simulink model "simulink_Cartpend_noControl"  (R2015a)
settings: Solver=ode45  StartTime=0.0  StopTime=10  MaxStep=0.01  RelTol=1e-3
undefined symbols (not defined in the file): bT, bX, g, L, mc, mp, y0
settings Model: Creator=Thomas  LastModifiedBy=Thomas
settings DataIOCC: ExternalInput=t  InitialState=yIn  SaveState=on

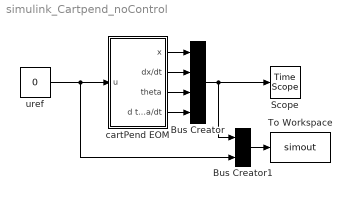
== system simulink_Cartpend_noControl ==
  Bus Creator : BusCreator
  Bus Creator1 : BusCreator  Inputs=2
  Scope : TimeScope
  To Workspace : ToWorkspace  VariableName=simout  SaveFormat=Structure With Time  SampleTime=-1
  cartPend EOM : Subsystem  mask(Inverted pendulum on cart){mc=mc, mp=mp, L=L, g=g, bX=bX, bT=bT}
      mask prompts: mc "Mass of cart (kg):"; mp "Mass of pendulum (kg):"; L "Distance to pendulum center of mass(m):"; g "Acceleration of gravity (m/s^2):"; bX "Damping of cart (kg/s)"; bT "Damping of pendulum (kg*m/s)"
      mask help: Unmask and double-click to see dynamics
      mask Help: Nonlinear dynamics of inverted pendulum on cart.
  uref : Constant  Value=0
  wires:
  Bus Creator/1 -> Scope/1, Bus Creator1/1
  cartPend EOM/4(d theta/dt) -> Bus Creator/4
  cartPend EOM/3("theta ") -> Bus Creator/3
  cartPend EOM/2(dx/dt) -> Bus Creator/2
  cartPend EOM/1(x) -> Bus Creator/1
  uref/1 -> Bus Creator1/2, cartPend EOM/1(u)
  Bus Creator1/1 -> To Workspace/1

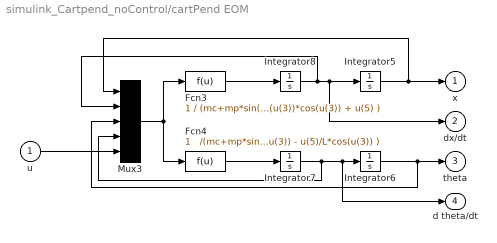
== system simulink_Cartpend_noControl/cartPend EOM ==
  u : Inport
  Fcn3 : Fcn  Expr="1 / (mc+mp*sin(u(3))^2)  * (   u(4)^2*mp*L*sin(u(3)) -u(4)*bT/L*cos(u(3))   -u(2)*bX  -   mp*g*sin(u(3))*cos(u(3)) + u(5) )"
  Fcn4 : Fcn  Expr="1   /(mc+mp*sin(u(3))^2)  * (   u(2)*bX/L*cos(u(3))   -   u(4)^2*mp*sin(u(3))*cos(u(3))   - u(4)*bT*(mc+mp)/ (L^2*mp)       + (mc+mp)*g/L*sin(u(3)) - u(5)/L*cos(u(3)) )"
  Integrator5 : Integrator  InitialCondition=y0(1)  ContinuousStateAttributes='x'
  Integrator6 : Integrator  InitialCondition=y0(3)  ContinuousStateAttributes='theta'
  Integrator7 : Integrator  InitialCondition=y0(4)  ContinuousStateAttributes='theta_dot'
  Integrator8 : Integrator  InitialCondition=y0(2)  ContinuousStateAttributes='xDot'
  Mux3 : Mux  Inputs=5
  x : Outport  InitialOutput=0
  dx/dt : Outport  Port=2  InitialOutput=0
  "theta " : Outport  Port=3  InitialOutput=0
  d theta/dt : Outport  Port=4  InitialOutput=0
  wires:
  Integrator5/1 -> Mux3/1, x/1
  Fcn4/1 -> Integrator7/1
  Mux3/1 -> Fcn3/1, Fcn4/1
  Fcn3/1 -> Integrator8/1
  Integrator8/1 -> Mux3/2, dx/dt/1, Integrator5/1
  Integrator7/1 -> Mux3/4, d theta/dt/1, Integrator6/1
  Integrator6/1 -> Mux3/3, "theta "/1
  u/1 -> Mux3/5
